simulink model "ACS_PIL"  (R2018b)
settings: Solver=FixedStepDiscrete  StartTime=0.0  StopTime=10000  FixedStep=0.01  MaxStep=10  RelTol=1e-5  AbsTol=1e-5  EnableMultiTasking=on
InitFcn:
  | initialization
values from neighbouring files (symbols this model uses):
  A = [0.25  0.25  0.25  0.25  0.25  0.25]    [initialization.m]
  AE = asin(Re/(Re+h))    [initialization.m]
  air_density = [1.2250e+000  3.8990e-002  1.7740e-002  8.2790e-003  3.9720e-003  1.9950e-003  1.0570e-003                5.8210e-004  3.2060e-004  1.7180e-004  8.7700e-005  4.1780e-005  1.9050e-005  8.3370e-006                3.3960e-006  1.3430e-006  5.2970e-007  9.6610e-008  2.4380e-008  8.4840e-009  3.8450e-009                2.0700e-009  1.2440e-009  5.4640e-010  2.7890e-010  7.2480e-011  2.4180e-011  9.1580 ...(+138 chars)    [initialization.m]
  altitude = [    0       25000       30000       35000       40000       45000       50000       55000             60000       65000       70000       75000       80000       85000       90000       95000            100000      110000      120000      130000      140000      150000      160000      180000            200000      250000      300000      350000      400000      450000      500000      600000     ...(+51 chars)    [initialization.m]
  c_diffus = [0.02   0.02   0.02    0.02    0.02    0.02]    [initialization.m]
  c_spec = [0.02   0.02   0.02    0.02    0.02    0.02]    [initialization.m]
  CD = 2    [initialization.m]
  Cell_Area = 30.18*1e-4    (= 0.003018)    [initialization.m]
  CM_mm01 = [-27723, 1088, -239;  -764, -25026, -219; 1299, -416, -23472]    [attitude_control.m]
  CM_mm02 = [-27799, 42,     95; -1261, -26308,  -43; 2693,  458, -24088]    [attitude_control.m]
  CM_mm03 = [9988,0,0; 0, 9989,0; 0,0,10036]    [attitude_control.m]
  CO_mm01 = [2.5332,  2.5200, 2.4915]    [attitude_control.m]
  CO_mm02 = [2.5348,  2.5260, 2.4664]    [attitude_control.m]
  CO_mm03 = [0.0008, -0.0006, 0.0007]    [attitude_control.m]
  cos50 = cos (50/360*2*pi)    [initialization.m]
  cosines = [0.087 0.174  0.500 0.634 0.866]    [initialization.m]
  dip_coel = acos(g01/H0)    [initialization.m]
  dip_long = atan2(h11,g11)    [initialization.m]
  E_EOL = E_BOL*TD_T*TD_R    (= 0.213003)    [initialization.m]
  H0 = norm([g01,g11,h11])    [initialization.m]
  inc = 1.7231    [initialization.m]
  Inertia_tensor = [2.8  0  0;                   0  2.8  0;                   0  0  2]    [initialization.m]
  K_l = 0.1    [initialization.m]
  kelly = [0.000 0.100  0.450 0.635 0.866]    [initialization.m]
  light_speed = 3e8    (= 300000000)    [initialization.m]
  M_SR = 1377*0.967    (= 1331.559)    [initialization.m]
  MM_Working = [1 1 0]    [attitude_control.m]
  N_B = [  1     0    0,         -1     0    0,          0     1    0,          0    -1    0,          0     0    1,          0     0   -1]    [initialization.m]
  Ncell_Xn = 40    [initialization.m]
  Ncell_Xp = 40    [initialization.m]
  Ncell_Yn = 40    [initialization.m]
  Ncell_Yp = 40    [initialization.m]
  Ncell_Zn = 00    (= 0)    [initialization.m]
  Ncell_Zp = 20    [initialization.m]
  NX = [1 0 0]    [initialization.m]
  NY = [0 1 0]    [initialization.m]
  NZ = [0 0 1]    [initialization.m]
  omega_BI_B0 = [0.1;-0.1;-0.1]    [initialization.m]
  omega_e = 7.29e-5    (= 7.29e-05)    [initialization.m]
  omega_o = (1/r)*(G*M/r)^0.5    (= 0.00108253225434)    [initialization.m]
  quat_0 = E321_to_quat([phi0, theta0, psi0])    [initialization.m]
  r = h + Re    (= 6978137)    [initialization.m]
  r_cm_B = [(0.156e-2 * 42.3 + 0.16917 * 22)/64.3,           (0.248e-1 * 42.3 + -0.35948e-1 * 22)/64.3,           (0.164e-2 * 42.3 + 0.14518e-3 * 22)/64.3]    [initialization.m]
  r_cp_a_B = [0 0 0]    [initialization.m]
  r_cp_s_B = [0 0 0]    [initialization.m]
  RAAN_rt = 2.02e-7    (= 2.02e-07)    [initialization.m]
  Re = 6378137    [initialization.m]
  t0 = 2456738.000000    (= 2456738)    [initialization.m]
  TA_0 = 0    [initialization.m]
  theta_g0 = 0    [initialization.m]
undefined symbols (not defined in the file or in its folder): DiscIntNeverNeededParam, magnitude, serial
libraries: simulink x15, vrlib x3, instrumentlib x3, realtime_pacer_lib x1
(part 3 of 3)

== system ACS_PIL/UPMSat_2/Solar_Panels/Power/factor of view X ==
  cos (fi) : Inport
  Abs1 : Abs
  Compare to cos (50) : simulink/Logic and Bit Operations/Compare To Constant  relop=>=  const=cos50  OutDataTypeStr=uint8  ZeroCross=off
  Kelly Cosine1 : Lookup  InputValues=cosines  Table=kelly
  Logical Operator : Logic  Operator=NOT  AllPortsSameDT=off  OutDataTypeStr=boolean
  Product : Product  RndMeth=Zero
  Product1 : Product  RndMeth=Zero
  Product2 : Product  RndMeth=Zero
  Saturation : Saturate  UpperLimit=1  LowerLimit=0
  Sign : Signum
  Sum : Sum
  FV : Outport
  wires:
  Sign/1 -> Product2/1
  Product2/1 -> FV/1
  Abs1/1 -> Compare to cos (50)/1, Kelly Cosine1/1, Product/1
  Saturation/1 -> Product1/2
  Kelly Cosine1/1 -> Saturation/1
  Product1/1 -> Sum/2
  Product/1 -> Sum/1
  Logical Operator/1 -> Product1/1
  Sum/1 -> Product2/2
  cos (fi)/1 -> Sign/1, Abs1/1
  Compare to cos (50)/1 -> Logical Operator/1, Product/2

== system ACS_PIL/UPMSat_2/Solar_Panels/Power/factor of view Y ==
  cos (fi) : Inport
  Abs1 : Abs
  Compare to cos (50) : simulink/Logic and Bit Operations/Compare To Constant  relop=>=  const=cos50  OutDataTypeStr=uint8  ZeroCross=off
  Kelly Cosine1 : Lookup  InputValues=cosines  Table=kelly
  Logical Operator : Logic  Operator=NOT  AllPortsSameDT=off  OutDataTypeStr=boolean
  Product : Product  RndMeth=Zero
  Product1 : Product  RndMeth=Zero
  Product2 : Product  RndMeth=Zero
  Saturation : Saturate  UpperLimit=1  LowerLimit=0
  Sign : Signum
  Sum : Sum
  FV : Outport
  wires:
  Compare to cos (50)/1 -> Product/2, Logical Operator/1
  cos (fi)/1 -> Abs1/1, Sign/1
  Sum/1 -> Product2/2
  Logical Operator/1 -> Product1/1
  Product/1 -> Sum/1
  Product1/1 -> Sum/2
  Kelly Cosine1/1 -> Saturation/1
  Saturation/1 -> Product1/2
  Abs1/1 -> Product/1, Kelly Cosine1/1, Compare to cos (50)/1
  Product2/1 -> FV/1
  Sign/1 -> Product2/1

== system ACS_PIL/UPMSat_2/Solar_Panels/Power/factor of view Z ==
  cos (fi) : Inport
  Abs1 : Abs
  Compare to cos (50) : simulink/Logic and Bit Operations/Compare To Constant  relop=>=  const=cos50  OutDataTypeStr=uint8  ZeroCross=off
  Kelly Cosine1 : Lookup  InputValues=cosines  Table=kelly
  Logical Operator : Logic  Operator=NOT  AllPortsSameDT=off  OutDataTypeStr=boolean
  Product : Product  RndMeth=Zero
  Product1 : Product  RndMeth=Zero
  Product2 : Product  RndMeth=Zero
  Saturation : Saturate  UpperLimit=1  LowerLimit=0
  Sign : Signum
  Sum : Sum
  FV : Outport
  wires:
  Sign/1 -> Product2/1
  Product2/1 -> FV/1
  Abs1/1 -> Compare to cos (50)/1, Kelly Cosine1/1, Product/1
  Saturation/1 -> Product1/2
  Kelly Cosine1/1 -> Saturation/1
  Product1/1 -> Sum/2
  Product/1 -> Sum/1
  Logical Operator/1 -> Product1/1
  Sum/1 -> Product2/2
  cos (fi)/1 -> Sign/1, Abs1/1
  Compare to cos (50)/1 -> Logical Operator/1, Product/2

== system ACS_PIL/UPMSat_2/Solar_Panels/Power/norm ==
  1 : Inport
  Add1 : Sum  Inputs=+
  Math Function2 : Math  Operator=square  SaturateOnIntegerOverflow=on
  Math Function3 : Math  Operator=sqrt  SaturateOnIntegerOverflow=on
  Product1 : Product  Inputs=*/  RndMeth=Zero
  2 : Outport
  wires:
  1/1 -> Math Function2/1, Product1/1
  Math Function3/1 -> Product1/2
  Add1/1 -> Math Function3/1
  Math Function2/1 -> Add1/1
  Product1/1 -> 2/1

== system ACS_PIL/UPMSat_2/Solar_Panels/Power/norm1 ==
  1 : Inport
  Add1 : Sum  Inputs=+
  Math Function2 : Math  Operator=square  SaturateOnIntegerOverflow=on
  Math Function3 : Math  Operator=sqrt  SaturateOnIntegerOverflow=on
  Product1 : Product  Inputs=*/  RndMeth=Zero
  2 : Outport
  wires:
  Product1/1 -> 2/1
  Math Function2/1 -> Add1/1
  Add1/1 -> Math Function3/1
  Math Function3/1 -> Product1/2
  1/1 -> Product1/1, Math Function2/1

== system ACS_PIL/UPMSat_2/Solar_Panels/Power/norm2 ==
  1 : Inport
  Add1 : Sum  Inputs=+
  Math Function2 : Math  Operator=square  SaturateOnIntegerOverflow=on
  Math Function3 : Math  Operator=sqrt  SaturateOnIntegerOverflow=on
  Product1 : Product  Inputs=*/  RndMeth=Zero
  2 : Outport
  wires:
  Product1/1 -> 2/1
  Math Function2/1 -> Add1/1
  Add1/1 -> Math Function3/1
  Math Function3/1 -> Product1/2
  1/1 -> Product1/1, Math Function2/1

== system ACS_PIL/UPMSat_2/Solar_Panels/Power/norm3 ==
  1 : Inport
  Add1 : Sum  Inputs=+
  Math Function2 : Math  Operator=square  SaturateOnIntegerOverflow=on
  Math Function3 : Math  Operator=sqrt  SaturateOnIntegerOverflow=on
  Product1 : Product  Inputs=*/  RndMeth=Zero
  2 : Outport
  wires:
  1/1 -> Math Function2/1, Product1/1
  Math Function3/1 -> Product1/2
  Add1/1 -> Math Function3/1
  Math Function2/1 -> Add1/1
  Product1/1 -> 2/1

== system ACS_PIL/UPMSat_2/Solar_Panels/Power/norm4 ==
  1 : Inport
  Add1 : Sum  Inputs=+
  Math Function2 : Math  Operator=square  SaturateOnIntegerOverflow=on
  Math Function3 : Math  Operator=sqrt  SaturateOnIntegerOverflow=on
  Product1 : Product  Inputs=*/  RndMeth=Zero
  2 : Outport
  wires:
  Product1/1 -> 2/1
  Math Function2/1 -> Add1/1
  Add1/1 -> Math Function3/1
  Math Function3/1 -> Product1/2
  1/1 -> Product1/1, Math Function2/1

== system ACS_PIL/UPMSat_2/Solar_Panels/Power/norm5 ==
  1 : Inport
  Add1 : Sum  Inputs=+
  Math Function2 : Math  Operator=square  SaturateOnIntegerOverflow=on
  Math Function3 : Math  Operator=sqrt  SaturateOnIntegerOverflow=on
  Product1 : Product  Inputs=*/  RndMeth=Zero
  2 : Outport
  wires:
  1/1 -> Math Function2/1, Product1/1
  Math Function3/1 -> Product1/2
  Add1/1 -> Math Function3/1
  Math Function2/1 -> Add1/1
  Product1/1 -> 2/1

== system ACS_PIL/Earth/Simple model of Earth's Magnetic Field1/Simple model of Earth's Magnetic Field1/Simple Magnetc Field/Earths magnetic field in Inertial frame1 ==
  R_ECEF : Inport
  dd_ECEF : Inport  Port=2
  TS : Inport  Port=3
  Divide : Product  Inputs=*/
  Divide1 : Product  Inputs=***
  Divide5 : Product  Inputs=**
  Divide6 : Product  Inputs=*/
  Dot Product : DotProduct  InputSameDT=on  OutDataTypeStr=Inherit: Inherit via internal rule
  If : If  IfExpression=(u1 > eps | u1 < -eps)
  If Action Subsystem : Subsystem  TreatAsAtomicUnit=on
  If Action Subsystem1 : Subsystem  TreatAsAtomicUnit=on
  Math Function : Math  Operator=pow  SaturateOnIntegerOverflow=on
  Merge : Merge
  Sum : Sum  Inputs=+-
  magnetic_field8 : ToWorkspace  VariableName=Rdotm  SampleTime=-1
  sat distance from Earth's CM3 : Constant  Value=r
  sat distance from Earth's CM : Constant  Value=r
  sat distance from Earth's CM1 : Constant  Value=3
  sat distance from Earth's CM3 : Constant  Value=3
  B_ECEF : Outport
  wires:
  Sum/1 -> Divide5/2
  dd_ECEF/1 -> Sum/2, Dot Product/2
  Divide6/1 -> Divide1/1, Dot Product/1
  sat distance from Earth's CM3/1 -> Divide6/2
  R_ECEF/1 -> Divide6/1
  TS/1 -> Divide/1
  sat distance from Earth's CM/1 -> Math Function/1
  sat distance from Earth's CM1/1 -> Math Function/2
  Math Function/1 -> Divide/2
  Divide/1 -> Divide5/1
  Divide5/1 -> B_ECEF/1
  sat distance from Earth's CM3/1 -> Divide1/2
  Divide1/1 -> Sum/1
  If/1 -> If Action Subsystem/Action
  If Action Subsystem/1(Out1) -> Merge/1
  Merge/1 -> magnetic_field8/1, Divide1/3
  If Action Subsystem1/1(Out1) -> Merge/2
  If/2 -> If Action Subsystem1/Action
  Dot Product/1 -> If/1, If Action Subsystem/1(In1)

== system ACS_PIL/Perturbations/perturbation_Torque1/Solar Torque and Force Calculation/Force_toque1/force on X+ ==
  P : Inport
  A_xp : Inport  Port=2
  theta_xp : Inport  Port=3
  C_S : Inport  Port=4
  C_D : Inport  Port=5
  S_ES_B : Inport  Port=6
  Constant : Constant
  Divide{1..2,4..5} (4 alike) : Product
  Divide3 : Product  Inputs=***
  Gain : Gain  Gain=1/3
  Gain1 : Gain  Gain=2
  Gain2 : Gain  Gain=-1
  Normal : Constant  Value=[1 0 0]
  Saturation : Saturate  UpperLimit=1  LowerLimit=0
  Sum : Sum  Inputs=+-
  Sum1 : Sum
  Sum2 : Sum  Inputs=2
  Trigonometric Function1 : Trigonometry  Operator=cos
  F_s_xp : Outport
  wires:
  Saturation/1 -> Divide3/1, Divide1/2
  Divide5/1 -> F_s_xp/1
  Sum2/1 -> Divide5/2
  Divide4/1 -> Sum2/1
  S_ES_B/1 -> Divide4/1
  Divide2/1 -> Sum2/2
  Normal/1 -> Divide2/2
  Gain1/1 -> Divide2/1
  Sum1/1 -> Gain1/1
  Gain/1 -> Sum1/2
  Divide1/1 -> Sum1/1
  C_D/1 -> Gain/1
  Sum/1 -> Divide4/2
  C_S/1 -> Divide1/1, Sum/2
  Constant/1 -> Sum/1
  theta_xp/1 -> Trigonometric Function1/1
  Trigonometric Function1/1 -> Saturation/1
  P/1 -> Divide3/2
  A_xp/1 -> Divide3/3
  Divide3/1 -> Gain2/1
  Gain2/1 -> Divide5/1

== system ACS_PIL/Perturbations/perturbation_Torque1/Solar Torque and Force Calculation/Force_toque1/force on X- ==
  P : Inport
  A_xm : Inport  Port=2
  theta_xm : Inport  Port=3
  C_S : Inport  Port=4
  C_D : Inport  Port=5
  S_ES_B : Inport  Port=6
  Constant : Constant
  Divide{1..2,4..5} (4 alike) : Product
  Divide3 : Product  Inputs=***
  Gain : Gain  Gain=1/3
  Gain1 : Gain  Gain=2
  Gain2 : Gain  Gain=-1
  Normal : Constant  Value=[-1 0 0]
  Saturation : Saturate  UpperLimit=1  LowerLimit=0
  Sum : Sum  Inputs=+-
  Sum1 : Sum
  Sum2 : Sum  Inputs=2
  Trigonometric Function1 : Trigonometry  Operator=cos
  F_s_xm : Outport
  wires:
  Gain2/1 -> Divide5/1
  Divide3/1 -> Gain2/1
  A_xm/1 -> Divide3/3
  P/1 -> Divide3/2
  Trigonometric Function1/1 -> Saturation/1
  theta_xm/1 -> Trigonometric Function1/1
  Constant/1 -> Sum/1
  C_S/1 -> Sum/2, Divide1/1
  Sum/1 -> Divide4/2
  C_D/1 -> Gain/1
  Divide1/1 -> Sum1/1
  Gain/1 -> Sum1/2
  Sum1/1 -> Gain1/1
  Gain1/1 -> Divide2/1
  Normal/1 -> Divide2/2
  Divide2/1 -> Sum2/2
  S_ES_B/1 -> Divide4/1
  Divide4/1 -> Sum2/1
  Sum2/1 -> Divide5/2
  Divide5/1 -> F_s_xm/1
  Saturation/1 -> Divide1/2, Divide3/1

== system ACS_PIL/Perturbations/perturbation_Torque1/Solar Torque and Force Calculation/Force_toque1/force on Y+ ==
  P : Inport
  A_yp : Inport  Port=2
  theta_yp : Inport  Port=3
  C_S : Inport  Port=4
  C_D : Inport  Port=5
  S_ES_B : Inport  Port=6
  Constant : Constant
  Divide{1..2,4..5} (4 alike) : Product
  Divide3 : Product  Inputs=***
  Gain : Gain  Gain=1/3
  Gain1 : Gain  Gain=2
  Gain2 : Gain  Gain=-1
  Normal : Constant  Value=[0 1 0]
  Saturation : Saturate  UpperLimit=1  LowerLimit=0
  Sum : Sum  Inputs=+-
  Sum1 : Sum
  Sum2 : Sum  Inputs=2
  Trigonometric Function1 : Trigonometry  Operator=cos
  F_s_yp : Outport
  wires:
  Saturation/1 -> Divide3/1, Divide1/2
  Divide5/1 -> F_s_yp/1
  Sum2/1 -> Divide5/2
  Divide4/1 -> Sum2/1
  S_ES_B/1 -> Divide4/1
  Divide2/1 -> Sum2/2
  Normal/1 -> Divide2/2
  Gain1/1 -> Divide2/1
  Sum1/1 -> Gain1/1
  Gain/1 -> Sum1/2
  Divide1/1 -> Sum1/1
  C_D/1 -> Gain/1
  Sum/1 -> Divide4/2
  C_S/1 -> Divide1/1, Sum/2
  Constant/1 -> Sum/1
  theta_yp/1 -> Trigonometric Function1/1
  Trigonometric Function1/1 -> Saturation/1
  P/1 -> Divide3/2
  A_yp/1 -> Divide3/3
  Divide3/1 -> Gain2/1
  Gain2/1 -> Divide5/1

== system ACS_PIL/Perturbations/perturbation_Torque1/Solar Torque and Force Calculation/Force_toque1/force on Y- ==
  P : Inport
  A_ym : Inport  Port=2
  theta_ym : Inport  Port=3
  C_S : Inport  Port=4
  C_D : Inport  Port=5
  S_ES_B : Inport  Port=6
  Constant : Constant
  Divide{1..2,4..5} (4 alike) : Product
  Divide3 : Product  Inputs=***
  Gain : Gain  Gain=1/3
  Gain1 : Gain  Gain=2
  Gain2 : Gain  Gain=-1
  Normal : Constant  Value=[0 -1 0]
  Saturation : Saturate  UpperLimit=1  LowerLimit=0
  Sum : Sum  Inputs=+-
  Sum1 : Sum
  Sum2 : Sum  Inputs=2
  Trigonometric Function1 : Trigonometry  Operator=cos
  F_s_ym : Outport
  wires:
  Saturation/1 -> Divide3/1, Divide1/2
  Divide5/1 -> F_s_ym/1
  Sum2/1 -> Divide5/2
  Divide4/1 -> Sum2/1
  S_ES_B/1 -> Divide4/1
  Divide2/1 -> Sum2/2
  Normal/1 -> Divide2/2
  Gain1/1 -> Divide2/1
  Sum1/1 -> Gain1/1
  Gain/1 -> Sum1/2
  Divide1/1 -> Sum1/1
  C_D/1 -> Gain/1
  Sum/1 -> Divide4/2
  C_S/1 -> Divide1/1, Sum/2
  Constant/1 -> Sum/1
  theta_ym/1 -> Trigonometric Function1/1
  Trigonometric Function1/1 -> Saturation/1
  P/1 -> Divide3/2
  A_ym/1 -> Divide3/3
  Divide3/1 -> Gain2/1
  Gain2/1 -> Divide5/1

== system ACS_PIL/Perturbations/perturbation_Torque1/Solar Torque and Force Calculation/Force_toque1/force on Z+ ==
  P : Inport
  A_zp : Inport  Port=2
  theta_zp : Inport  Port=3
  C_S : Inport  Port=4
  C_D : Inport  Port=5
  S_ES_B : Inport  Port=6
  Constant : Constant
  Divide{1..2,4..5} (4 alike) : Product
  Divide3 : Product  Inputs=***
  Gain : Gain  Gain=1/3
  Gain1 : Gain  Gain=2
  Gain2 : Gain  Gain=-1
  Normal : Constant  Value=[0 0 1]
  Saturation : Saturate  UpperLimit=1  LowerLimit=0
  Sum : Sum  Inputs=+-
  Sum1 : Sum
  Sum2 : Sum  Inputs=2
  Trigonometric Function1 : Trigonometry  Operator=cos
  F_s_zp : Outport
  wires:
  Gain2/1 -> Divide5/1
  Divide3/1 -> Gain2/1
  A_zp/1 -> Divide3/3
  P/1 -> Divide3/2
  Trigonometric Function1/1 -> Saturation/1
  theta_zp/1 -> Trigonometric Function1/1
  Constant/1 -> Sum/1
  C_S/1 -> Sum/2, Divide1/1
  Sum/1 -> Divide4/2
  C_D/1 -> Gain/1
  Divide1/1 -> Sum1/1
  Gain/1 -> Sum1/2
  Sum1/1 -> Gain1/1
  Gain1/1 -> Divide2/1
  Normal/1 -> Divide2/2
  Divide2/1 -> Sum2/2
  S_ES_B/1 -> Divide4/1
  Divide4/1 -> Sum2/1
  Sum2/1 -> Divide5/2
  Divide5/1 -> F_s_zp/1
  Saturation/1 -> Divide1/2, Divide3/1

== system ACS_PIL/Perturbations/perturbation_Torque1/Solar Torque and Force Calculation/Force_toque1/force on Z- ==
  P : Inport
  A_zm : Inport  Port=2
  theta_zm : Inport  Port=3
  C_S : Inport  Port=4
  C_D : Inport  Port=5
  S_ES_B : Inport  Port=6
  Constant : Constant
  Divide{1..2,4..5} (4 alike) : Product
  Divide3 : Product  Inputs=***
  Gain : Gain  Gain=1/3
  Gain1 : Gain  Gain=2
  Gain2 : Gain  Gain=-1
  Normal : Constant  Value=[0 0 -1]
  Saturation : Saturate  UpperLimit=1  LowerLimit=0
  Sum : Sum  Inputs=+-
  Sum1 : Sum
  Sum2 : Sum  Inputs=2
  Trigonometric Function1 : Trigonometry  Operator=cos
  F_s_zm : Outport
  wires:
  Saturation/1 -> Divide3/1, Divide1/2
  Divide5/1 -> F_s_zm/1
  Sum2/1 -> Divide5/2
  Divide4/1 -> Sum2/1
  S_ES_B/1 -> Divide4/1
  Divide2/1 -> Sum2/2
  Normal/1 -> Divide2/2
  Gain1/1 -> Divide2/1
  Sum1/1 -> Gain1/1
  Gain/1 -> Sum1/2
  Divide1/1 -> Sum1/1
  C_D/1 -> Gain/1
  Sum/1 -> Divide4/2
  C_S/1 -> Divide1/1, Sum/2
  Constant/1 -> Sum/1
  theta_zm/1 -> Trigonometric Function1/1
  Trigonometric Function1/1 -> Saturation/1
  P/1 -> Divide3/2
  A_zm/1 -> Divide3/3
  Divide3/1 -> Gain2/1
  Gain2/1 -> Divide5/1

== system ACS_PIL/UPMSat_2/OBC/Nominal Attitude Control/Sensor/Average ==
  B_b_T : Inport
  MM_working : Inport  Port=2
  Bus Selector : BusSelector  OutputSignals=B_MM1,B_MM2,B_MM3
  Demux : Demux  Outputs=3
  Product : Product
  Product1 : Product
  Product2 : Product
  Product3 : Product  Inputs=*/
  Sum : Sum  Inputs=3
  Sum of Elements : Sum  Inputs=+
  B_b_T_1s : Outport
  wires:
  MM_working/1 -> Demux/1, Sum of Elements/1
  Demux/1 -> Product/2  "MM1_working"
  Demux/2 -> Product1/2  "MM2_working"
  Demux/3 -> Product2/2  "MM3_Working"
  Product/1 -> Sum/1
  Product1/1 -> Sum/2
  Product2/1 -> Sum/3
  Sum/1 -> Product3/1
  Product3/1 -> B_b_T_1s/1
  Sum of Elements/1 -> Product3/2
  B_b_T/1 -> Bus Selector/1
  Bus Selector/1 -> Product/1  "<B_MM1>"
  Bus Selector/2 -> Product1/1  "<B_MM2>"
  Bus Selector/3 -> Product2/1  "<B_MM3>"

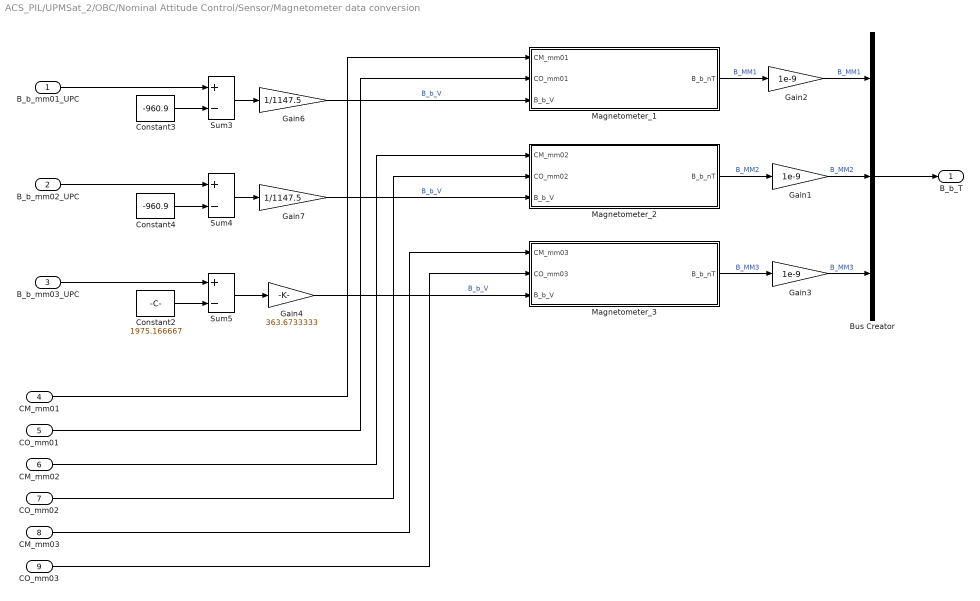
== system ACS_PIL/UPMSat_2/OBC/Nominal Attitude Control/Sensor/Magnetometer data conversion  ==
  B_b_mm01_UPC : Inport
  B_b_mm02_UPC : Inport  Port=2
  B_b_mm03_UPC : Inport  Port=3
  CM_mm01 : Inport  Port=4
  CO_mm01 : Inport  Port=5
  CM_mm02 : Inport  Port=6
  CO_mm02 : Inport  Port=7
  CM_mm03 : Inport  Port=8
  CO_mm03 : Inport  Port=9
  Bus Creator : BusCreator  Inputs=3
  Constant2 : Constant  Value=1975.166667  OutDataTypeStr=single
  Constant3 : Constant  Value=-960.9  OutDataTypeStr=single
  Constant4 : Constant  Value=-960.9  OutDataTypeStr=single
  Gain1 : Gain  Gain=1e-9
  Gain2 : Gain  Gain=1e-9
  Gain3 : Gain  Gain=1e-9
  Gain4 : Gain  Gain=363.6733333
  Gain6 : Gain  Gain=1/1147.5
  Gain7 : Gain  Gain=1/1147.5
  Magnetometer_1 : Subsystem
  Magnetometer_2 : Subsystem
  Magnetometer_3 : Subsystem
  Sum3 : Sum  Inputs=+-
  Sum4 : Sum  Inputs=+-
  Sum5 : Sum  Inputs=+-
  B_b_T : Outport
  wires:
  Magnetometer_1/1(B_b_nT) -> Gain2/1  "B_MM1"
  Magnetometer_2/1(B_b_nT) -> Gain1/1  "B_MM2"
  B_b_mm02_UPC/1 -> Sum4/1
  Bus Creator/1 -> B_b_T/1
  Gain2/1 -> Bus Creator/1  "B_MM1"
  Gain1/1 -> Bus Creator/2  "B_MM2"
  Gain3/1 -> Bus Creator/3  "B_MM3"
  B_b_mm03_UPC/1 -> Sum5/1
  Magnetometer_3/1(B_b_nT) -> Gain3/1  "B_MM3"
  B_b_mm01_UPC/1 -> Sum3/1
  Sum3/1 -> Gain6/1
  Sum4/1 -> Gain7/1
  Sum5/1 -> Gain4/1
  Gain6/1 -> Magnetometer_1/3(B_b_V)  "B_b_V"
  Gain7/1 -> Magnetometer_2/3(B_b_V)  "B_b_V"
  Gain4/1 -> Magnetometer_3/3(B_b_V)  "B_b_V"
  Constant3/1 -> Sum3/2
  Constant4/1 -> Sum4/2
  Constant2/1 -> Sum5/2
  CM_mm01/1 -> Magnetometer_1/1(CM_mm01)
  CO_mm01/1 -> Magnetometer_1/2(CO_mm01)
  CM_mm02/1 -> Magnetometer_2/1(CM_mm02)
  CO_mm02/1 -> Magnetometer_2/2(CO_mm02)
  CM_mm03/1 -> Magnetometer_3/1(CM_mm03)
  CO_mm03/1 -> Magnetometer_3/2(CO_mm03)

== system ACS_PIL/UPMSat_2/OBC/Nominal Attitude Control/Sensor/Memory ==
  B_b_T : Inport
  Mux : Mux  Inputs=5
  Terminator : Terminator
  Unit Delay{,1..4} (5 alike) : UnitDelay  SampleTime=-1
  B_b_T_1s : Outport
  wires:
  Unit Delay4/1 -> Terminator/1, Mux/5
  Mux/1 -> B_b_T_1s/1
  Unit Delay3/1 -> Unit Delay4/1, Mux/4
  Unit Delay2/1 -> Unit Delay3/1, Mux/3
  Unit Delay1/1 -> Unit Delay2/1, Mux/2
  Unit Delay/1 -> Unit Delay1/1, Mux/1
  B_b_T/1 -> Unit Delay/1

== system ACS_PIL/Earth/Simple model of Earth's Magnetic Field1/Simple model of Earth's Magnetic Field1/Simple Magnetc Field/Earths magnetic field in Inertial frame1/If Action Subsystem ==
  In1 : Inport
  Action Port : ActionPort  ActionType=then
  Out1 : Outport
  wires:
  In1/1 -> Out1/1

== system ACS_PIL/Earth/Simple model of Earth's Magnetic Field1/Simple model of Earth's Magnetic Field1/Simple Magnetc Field/Earths magnetic field in Inertial frame1/If Action Subsystem1 ==
  Action Port : ActionPort  ActionType=else
  sat distance from Earth's CM3 : Constant  Value=0
  Out1 : Outport
  wires:
  sat distance from Earth's CM3/1 -> Out1/1

== system ACS_PIL/UPMSat_2/OBC/Nominal Attitude Control/Sensor/Magnetometer data conversion /Magnetometer_1 ==
  CM_mm01 : Inport
  CO_mm01 : Inport  Port=2
  B_b_V : Inport  Port=3
  Product : Product  Multiplication=Matrix(*)  RndMeth=Zero
  Sum : Sum  Inputs=-+
  B_b_nT : Outport
  wires:
  B_b_V/1 -> Sum/2
  Sum/1 -> Product/2
  Product/1 -> B_b_nT/1
  CO_mm01/1 -> Sum/1
  CM_mm01/1 -> Product/1

== system ACS_PIL/UPMSat_2/OBC/Nominal Attitude Control/Sensor/Magnetometer data conversion /Magnetometer_2 ==
  CM_mm02 : Inport
  CO_mm02 : Inport  Port=2
  B_b_V : Inport  Port=3
  Product : Product  Multiplication=Matrix(*)  RndMeth=Zero
  Sum : Sum  Inputs=-+
  B_b_nT : Outport
  wires:
  B_b_V/1 -> Sum/2
  Sum/1 -> Product/2
  Product/1 -> B_b_nT/1
  CM_mm02/1 -> Product/1
  CO_mm02/1 -> Sum/1

== system ACS_PIL/UPMSat_2/OBC/Nominal Attitude Control/Sensor/Magnetometer data conversion /Magnetometer_3 ==
  CM_mm03 : Inport
  CO_mm03 : Inport  Port=2
  B_b_V : Inport  Port=3
  Product : Product  Multiplication=Matrix(*)  RndMeth=Zero
  Sum : Sum  Inputs=-+
  B_b_nT : Outport
  wires:
  B_b_V/1 -> Sum/2
  Sum/1 -> Product/2
  Product/1 -> B_b_nT/1
  CO_mm03/1 -> Sum/1
  CM_mm03/1 -> Product/1
